simulink subsystem "NPC"  (R2021a)
settings: Solver=VariableStepAuto  StartTime=0.0  StopTime=10.0  RelTol=1e-3
libraries: mpcadaslib x1, drivingvehiclecontroller x1, robotalgslib x1
settings Model: Creator=Avvienash  LastModifiedBy=Avvienash

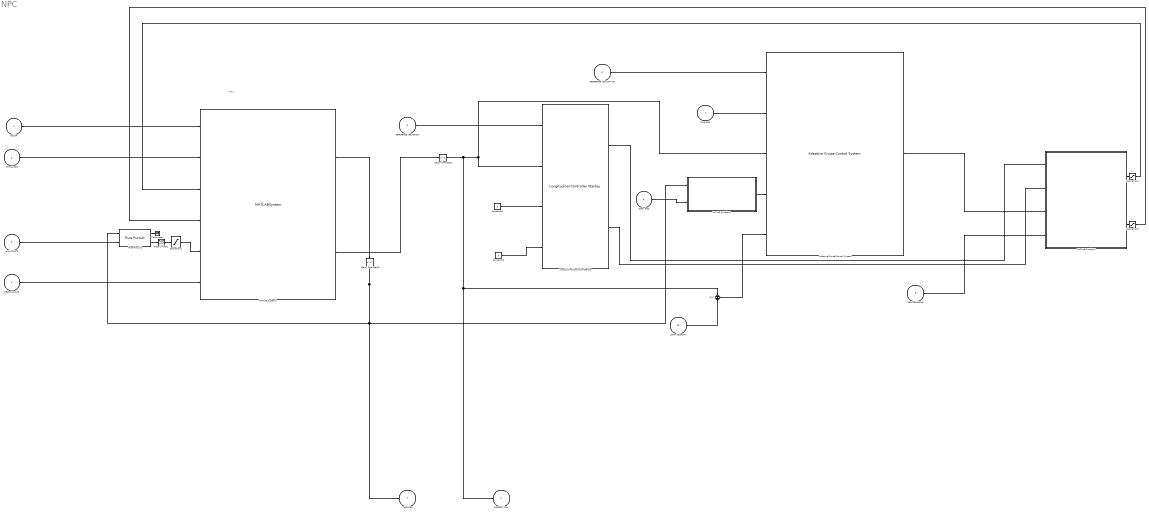
== system NPC ==
  note: NPC 1
  "COLOR " : Inport
  INITIAL POS : Inport  Port=2
  WAYPOINTS : Inport  Port=3
  RESPWAN POS : Inport  Port=4
  REFERENCE VEL CONST : Inport  Port=5
  REFERENCE VEL CATHUP : Inport  Port=6
  TIME GAP : Inport  Port=7
  LEAD BOOLEAN : Inport  Port=8
  LEAD  POS : Inport  Port=9
  LEAD VELOCITY : Inport  Port=10
  Adaptive Cruise Control System : mpcadaslib/Adaptive Cruise Control System  EgoModel=tf(1,[0.5,1,0])  InitialEgoVelocity=5  DefaultSpacing=2  MaxVelocity=20  MinAcceleration=-0.5  amin_ext=off  MaxAcceleration=1  amax_ext=off  Ts=0.05  PredictionHorizon=30  ControllerBehavior=0.520  suboptimal=off  maxiter=10  datatypeopt=double  optmode=off  trackmode=off
  Constant11 : Constant
  Constant12 : Constant  Value=0
  Delay One Step2 : Delay  DelayLength=1  InitialCondition=0
  Delay One Step3 : Delay  DelayLength=1  InitialCondition=[200 8.5 7.2]
  Longitudinal Controller Stanley : drivingvehiclecontroller/Longitudinal Controller Stanley  Kp=2.5  Ki=1  SampleTime=0.05  MaxAcceleration=1  MaxDeceleration=1
      settings: SourceProductBaseCode=DR
  MATLAB Function1 : MATLAB Function
  MATLAB Function2 : MATLAB Function
  MATLAB System1 : MATLABSystem  System=Traffic_NPC  SimulateUsing=Interpreted execution
      mask Type: Traffic_NPC
      mask Display:
      | disp('Traffic_NPC');
      | port_label('input',1,'color');
      | port_label('input',2,'init_pos');
      | port_label('input',3,'throttle');
      | port_label('input',4,'brake');
      | port_label('input',5,'steer');
      | port_label('input',6,'restart_pos');
      | port_label('output',1,'pos');
      | port_label('output',2,'long_velocity');
  Pure Pursuit1 : robotalgslib/Pure Pursuit  DesiredLinearVelocity=5  MaxAngularVelocity=1  LookaheadDistance=5  TargetDirPort=off  SimulateUsing=Code generation
  Rate Limiter1 : RateLimiter  SampleTimeMode=inherited
  Saturation1 : Saturate  UpperLimit=1  LowerLimit=-1
  Saturation4 : Saturate  UpperLimit=1  LowerLimit=0
  Saturation5 : Saturate  UpperLimit=1  LowerLimit=0
  Sum : Sum  Inputs=-|+
  Terminator : Terminator
  CURR POS : Outport
  CURRENT VEL : Outport  Port=2
  wires:
  Saturation1/1 -> MATLAB System1/5
  Longitudinal Controller Stanley/2 -> MATLAB Function2/2(dcc1)
  REFERENCE VEL CONST/1 -> Longitudinal Controller Stanley/1
  LEAD VELOCITY/1 -> Sum/2
  RESPWAN POS/1 -> MATLAB System1/6
  WAYPOINTS/1 -> Pure Pursuit1/2
  "COLOR "/1 -> MATLAB System1/1
  LEAD  POS/1 -> MATLAB Function1/2(lead_pos)
  MATLAB Function2/2(DCC) -> Saturation5/1
  REFERENCE VEL CATHUP/1 -> Adaptive Cruise Control System/1
  Adaptive Cruise Control System/1 -> MATLAB Function2/3(acc2)
  Saturation4/1 -> MATLAB System1/3
  Pure Pursuit1/2 -> Rate Limiter1/1
  Pure Pursuit1/1 -> Terminator/1
  Sum/1 -> Adaptive Cruise Control System/5
  Longitudinal Controller Stanley/1 -> MATLAB Function2/1(acc1)
  Delay One Step2/1 -> Sum/1, CURRENT VEL/1, Adaptive Cruise Control System/3, Longitudinal Controller Stanley/2
  Saturation5/1 -> MATLAB System1/4
  TIME GAP/1 -> Adaptive Cruise Control System/2
  MATLAB System1/2 -> Delay One Step2/1
  MATLAB Function1/1(y) -> Adaptive Cruise Control System/4
  MATLAB Function2/1(ACC) -> Saturation4/1
  LEAD BOOLEAN/1 -> MATLAB Function2/4(l)
  Rate Limiter1/1 -> Saturation1/1
  MATLAB System1/1 -> Delay One Step3/1
  INITIAL POS/1 -> MATLAB System1/2
  Constant12/1 -> Longitudinal Controller Stanley/4
  Constant11/1 -> Longitudinal Controller Stanley/3
  Delay One Step3/1 -> CURR POS/1, MATLAB Function1/1(pos), Pure Pursuit1/1

== matlab function NPC/MATLAB Function1 ==
  data: pos input; y output; lead_pos input
function y = fcn(pos,lead_pos)

y = -1*(lead_pos - pos(1)) - 2.4 ;

== matlab function NPC/MATLAB Function2 ==
  data: acc1 input; ACC output; dcc1 input; acc2 input; l input; DCC output
function [ACC,DCC] = fcn(acc1,dcc1,acc2,l)

    if l == 1
        ACC  = acc1;
        DCC = dcc1;
    else
        ACC  = acc2;
        DCC = -1*acc2;
    end
end
